simulink model "SVPWM_simple_10000"  (R2021b)
settings: Solver=ode3  StartTime=0.0  StopTime=1  FixedStep=1e-5  RelTol=1e-3
libraries: simulink x1, spspowerguiLib x1
settings Model: Creator=zyh  LastModifiedBy=zyh
settings SolverCC: AlgebraicLoopSolver=TrustRegion
settings DataIOCC: ReturnWorkspaceOutputs=off
settings DebuggingCC: MaskedZcDiagnostic=none  IgnoredZcDiagnostic=none  SFMachineParentedDataDiag=warning  ArithmeticOperatorsInVariantConditions=warning
settings SFSimCC: CustomCodeUndefinedFunction=UseInterfaceOnly

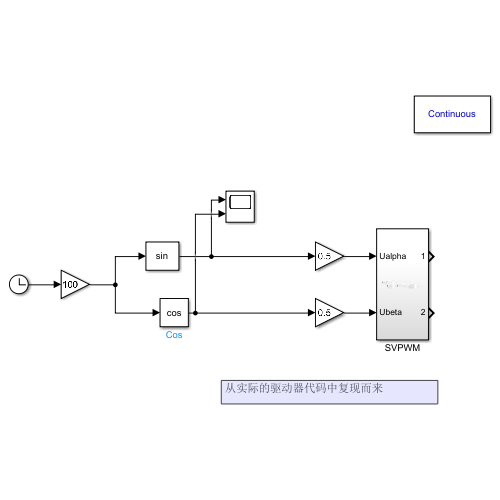
[thumbnail: Simulink's stored preview of the top-level diagram]
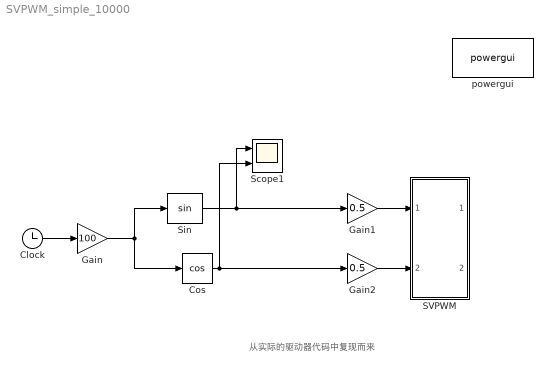
== system SVPWM_simple_10000 ==
  note: 从实际的驱动器代码中复现而来
  Clock : Clock
  Cos : Trigonometry  Operator=cos
  Gain : Gain  Gain=100
  Gain1 : Gain  Gain=0.5
  Gain2 : Gain  Gain=0.5
  SVPWM : Subsystem
  Scope1 : Scope  NumInputPorts=2
  Sin : Trigonometry
  powergui : spspowerguiLib/powergui  Priority=1  SimulationMode=Continuous  SampleTime=1e-6  frequency=60  Iterations=50  frequencyindice=0  Pbase=100e6  ErrMax=1e-4  UnitsV=kV  UnitsW=MW  buscounter=0  FunctionMessages=off  echomessages=off  EnableUseOfTLC=off  CurrentSourceSwitches=off  DisableSnubberDevices=off  DisableRonSwitches=off  DisableVfSwitches=off  DisplayEquations=off  AutomaticDiscreteSolvers=off  SolverType=Tustin/Backward Euler (TBE)  Interpol=off  ExternalGateDelay=off  methode=off  Ts=100  x0status=blocks  SPID=on  SwTol=0  HookPort=off  NonlinearTolerance=1e-4  nMaxIteration=100  ContinueOnMaxIteration=off  RestoreLinks=warning  ResistiveCurrentMeasurement=off  Frange=[0:2:500]  Ylog=off  Xlog=on  ShowGrid=off  save=off  variable=ZData  structure=0  ZoomFFT=off  StartTime=0.0  cycles=1  DisplayStyle=1  fundamental=60  FreqAxis=off  MaxFrequency=1000  frequencyindicesteady=1  RmsSteady=1  display=off
  wires:
  Cos/1 -> Gain2/1, Scope1/2
  Gain/1 -> Cos/1, Sin/1
  Clock/1 -> Gain/1
  Sin/1 -> Scope1/1, Gain1/1
  Gain1/1 -> SVPWM/1(Ualpha)
  Gain2/1 -> SVPWM/2(Ubeta)

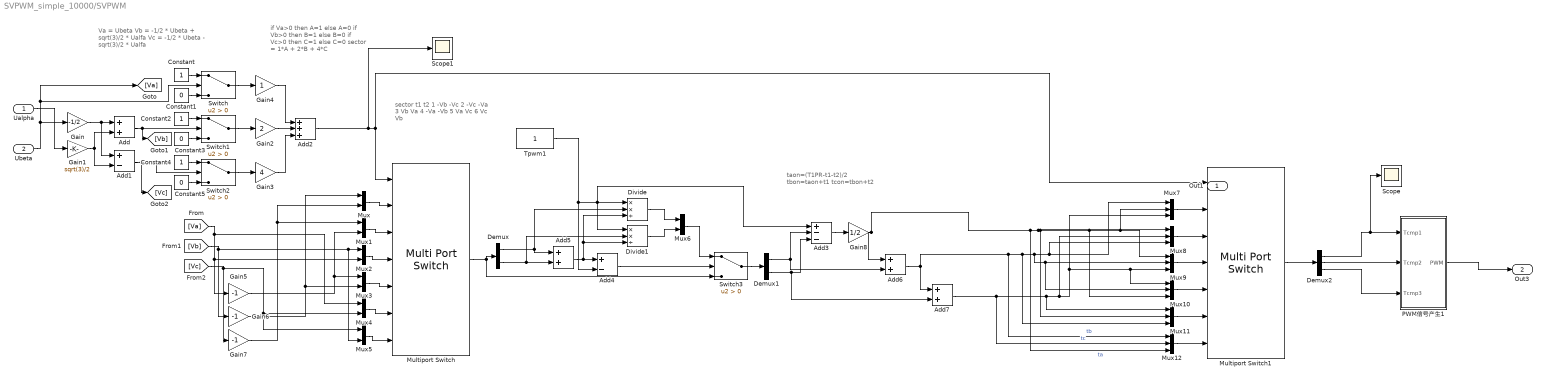
== system SVPWM_simple_10000/SVPWM ==
  note: taon=(T1PR-t1-t2)/2
      | tbon=taon+t1
      | tcon=tbon+t2
  note: sector   t1       t2
      | 1        -Vb     -Vc
      | 2        -Vc     -Va
      | 3         Vb      Va
      | 4        -Va     -Vb
      | 5         Va      Vc
      | 6         Vc      Vb
  note: if Va>0 then A=1 else A=0
      | if Vb>0 then B=1 else B=0
      | if Vc>0 then C=1 else C=0
      | sector = 1*A + 2*B + 4*C
  note: Va = Ubeta
      | Vb = -1/2 * Ubeta + sqrt(3)/2 * Ualfa
      | Vc = -1/2 * Ubeta - sqrt(3)/2 * Ualfa
  Ualpha : Inport
  Ubeta : Inport  Port=2
  Add{,5..7} (4 alike) : Sum
  Add1 : Sum  Inputs=+-
  Add2 : Sum  Inputs=+++
  Add3 : Sum  Inputs=+--
  Add4 : Sum  Inputs=+-
  Constant : Constant
  Constant1 : Constant  Value=0
  Constant2 : Constant
  Constant3 : Constant  Value=0
  Constant4 : Constant
  Constant5 : Constant  Value=0
  Demux : Demux  Outputs=2
  Demux1 : Demux  Outputs=2
  Demux2 : Demux  Outputs=3
  Divide : Product  Inputs=**/
  Divide1 : Product  Inputs=**/
  Gain : Gain  Gain=-1/2
  Gain1 : Gain  Gain=sqrt(3)/2
  Gain2 : Gain  Gain=2
  Gain3 : Gain  Gain=4
  Gain4 : Gain
  Gain5 : Gain  Gain=-1
  Gain6 : Gain  Gain=-1
  Gain7 : Gain  Gain=-1
  Gain8 : Gain  Gain=1/2
  Multiport Switch : MultiPortSwitch  Inputs=6  DiagnosticForDefault=None  OutDataTypeStr=double
  Multiport Switch1 : MultiPortSwitch  Inputs=6  DiagnosticForDefault=None  OutDataTypeStr=double
  Mux{,1..6} (7 alike) : Mux  Inputs=2
  Mux{7..12} (6 alike) : Mux  Inputs=3
  PWM信号产生1 : Subsystem
  Scope : Scope
  Scope1 : Scope
  Switch{,1..3} (4 alike) : Switch  Criteria=u2 > Threshold
  Tpwm1 : Constant
  Out1 : Outport  VectorParamsAs1DForOutWhenUnconnected=off
  Out3 : Outport  Port=2  VectorParamsAs1DForOutWhenUnconnected=off
  wires:
  Ualpha/1 -> Gain1/1
  Ubeta/1 -> Gain/1, Switch/2, [Va]
  Gain/1 -> Add1/1, Add/1
  Gain1/1 -> Add/2, Add1/2
  Add1/1 -> [Vc], Switch2/2
  Constant/1 -> Switch/1
  Constant1/1 -> Switch/3
  Constant3/1 -> Switch1/3
  Constant2/1 -> Switch1/1
  Add/1 -> [Vb], Switch1/2
  Constant4/1 -> Switch2/1
  Constant5/1 -> Switch2/3
  Switch1/1 -> Gain2/1
  Switch2/1 -> Gain3/1
  Switch/1 -> Gain4/1
  Gain4/1 -> Add2/1
  Gain2/1 -> Add2/2
  Gain3/1 -> Add2/3
  Add2/1 -> Scope1/1, Multiport Switch/1, Multiport Switch1/1
  [Va] -> Mux4/1, Mux2/2, Gain5/1
  [Vb] -> Mux5/2, Mux2/1, Gain6/1
  [Vc] -> Mux5/1, Mux4/2, Gain7/1
  Mux/1 -> Multiport Switch/2
  Gain6/1 -> Mux3/2, Mux/1
  Gain7/1 -> Mux/2, Mux1/1
  Gain5/1 -> Mux3/1, Mux1/2
  Mux1/1 -> Multiport Switch/3
  Mux2/1 -> Multiport Switch/4
  Mux3/1 -> Multiport Switch/5
  Mux4/1 -> Multiport Switch/6
  Mux5/1 -> Multiport Switch/7
  Multiport Switch/1 -> Demux/1, Switch3/3
  Demux/1 -> Add5/1, Divide/2
  Demux/2 -> Divide1/2, Add5/2
  Add5/1 -> Divide1/3, Divide/3, Add4/1
  Tpwm1/1 -> Add4/2, Add3/1, Divide1/1, Divide/1
  Add4/1 -> Switch3/2
  Divide/1 -> Mux6/1
  Divide1/1 -> Mux6/2
  Mux6/1 -> Switch3/1
  Switch3/1 -> Demux1/1
  Demux1/1 -> Add3/2, Add6/2
  Demux1/2 -> Add7/2, Add3/3
  Add3/1 -> Gain8/1
  Gain8/1 -> Mux12/3, Mux11/2, Mux10/3, Mux9/1, Mux7/2, Mux8/1, Add6/1  "ta"
  Add6/1 -> Mux12/1, Mux11/3, Mux10/2, Mux9/2, Mux8/3, Mux7/1, Add7/1  "tb"
  Add7/1 -> Mux12/2, Mux11/1, Mux8/2, Mux10/1, Mux9/3, Mux7/3  "tc"
  PWM信号产生1/1(PWM) -> Out3/1
  Mux7/1 -> Multiport Switch1/2
  Mux8/1 -> Multiport Switch1/3
  Mux9/1 -> Multiport Switch1/4
  Mux10/1 -> Multiport Switch1/5
  Mux11/1 -> Multiport Switch1/6
  Mux12/1 -> Multiport Switch1/7
  Multiport Switch1/1 -> Demux2/1
  Demux2/1 -> Scope/1, PWM信号产生1/1(Tcmp1)
  Demux2/2 -> PWM信号产生1/2(Tcmp2)
  Demux2/3 -> PWM信号产生1/3(Tcmp3)

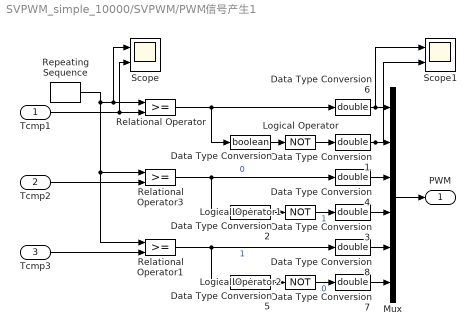
== system SVPWM_simple_10000/SVPWM/PWM信号产生1 ==
  Tcmp1 : Inport
  Tcmp2 : Inport  Port=2
  Tcmp3 : Inport  Port=3
  Data Type Conversion : DataTypeConversion  OutDataTypeStr=boolean
  Data Type Conversion{1,3..4,6..8} (6 alike) : DataTypeConversion  OutDataTypeStr=double
  Data Type Conversion2 : DataTypeConversion  OutDataTypeStr=boolean
  Data Type Conversion5 : DataTypeConversion  OutDataTypeStr=boolean
  Logical Operator : Logic  Operator=NOT  AllPortsSameDT=off  OutDataTypeStr=boolean
  Logical Operator1 : Logic  Operator=NOT  AllPortsSameDT=off  OutDataTypeStr=boolean
  Logical Operator2 : Logic  Operator=NOT  AllPortsSameDT=off  OutDataTypeStr=boolean
  Mux : Mux  Inputs=6
  Relational Operator : RelationalOperator  OutDataTypeStr=boolean  RndMeth=Nearest
  Relational Operator1 : RelationalOperator  OutDataTypeStr=boolean  RndMeth=Nearest
  Relational Operator3 : RelationalOperator  OutDataTypeStr=boolean  RndMeth=Nearest
  Repeating Sequence : simulink/Sources/Repeating Sequence  rep_seq_t=[0 1e-4 2e-4]  rep_seq_y=[0 1.3e-6 0]
  Scope : Scope  NumInputPorts=2
  Scope1 : Scope  NumInputPorts=2
  PWM : Outport  VectorParamsAs1DForOutWhenUnconnected=off
  wires:
  Data Type Conversion/1 -> Logical Operator/1
  Logical Operator/1 -> Data Type Conversion1/1
  Relational Operator/1 -> Data Type Conversion6/1, Data Type Conversion/1
  Logical Operator1/1 -> Data Type Conversion3/1  "1"
  Relational Operator3/1 -> Data Type Conversion4/1, Data Type Conversion2/1  "0"
  Data Type Conversion2/1 -> Logical Operator1/1
  Relational Operator1/1 -> Data Type Conversion8/1, Data Type Conversion5/1  "1"
  Data Type Conversion5/1 -> Logical Operator2/1
  Logical Operator2/1 -> Data Type Conversion7/1  "0"
  Repeating Sequence/1 -> Relational Operator1/1, Relational Operator3/1, Scope/1, Relational Operator/1
  Tcmp1/1 -> Scope/2, Relational Operator/2
  Tcmp2/1 -> Relational Operator3/2
  Tcmp3/1 -> Relational Operator1/2
  Data Type Conversion1/1 -> Scope1/2, Mux/2
  Data Type Conversion4/1 -> Mux/3
  Data Type Conversion3/1 -> Mux/4
  Data Type Conversion8/1 -> Mux/5
  Data Type Conversion7/1 -> Mux/6
  Mux/1 -> PWM/1
  Data Type Conversion6/1 -> Scope1/1, Mux/1
